simulink model "untitledlineal"  (R2014a)
settings: Solver=ode45  StartTime=0.0  StopTime=100  RelTol=1e-3
settings Model: Creator=Sec-E-B Ingenieria  LastModifiedBy=Sec-E-B Ingenieria

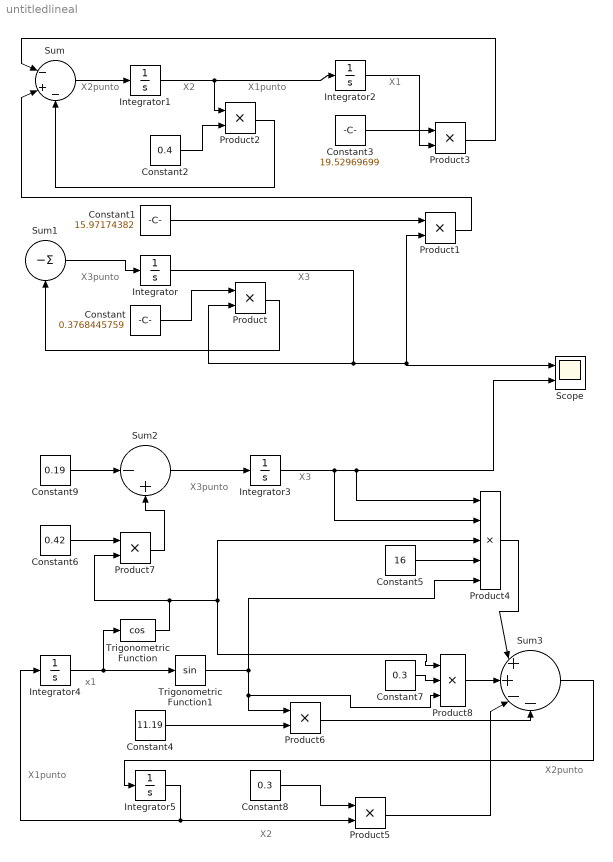
== system untitledlineal ==
  note: X3
  note: X3punto
  note: X1
  note: X1punto
  note: X2
  note: X2punto
  note: x1
  note: X1punto
  note: X2
  note: X2punto
  note: X3
  note: X3punto
  Constant : Constant  Value=0.3768445759
  Constant1 : Constant  Value=15.97174382
  Constant2 : Constant  Value=0.4
  Constant3 : Constant  Value=19.52969699
  Constant4 : Constant  Value=11.19
  Constant5 : Constant  Value=16
  Constant6 : Constant  Value=0.42
  Constant7 : Constant  Value=0.3
  Constant8 : Constant  Value=0.3
  Constant9 : Constant  Value=0.19
  Integrator : Integrator  InitialCondition=3
  Integrator1 : Integrator
  Integrator2 : Integrator
  Integrator3 : Integrator  InitialCondition=-1
  Integrator4 : Integrator  InitialCondition=1
  Integrator5 : Integrator
  Product{,1..3,5..7} (7 alike) : Product
  Product4 : Product  Inputs=5  InputSameDT=on
  Product8 : Product  Inputs=3
  Scope : Scope  NumInputPorts=2
      settings: YMin=-5~-5  YMax=5~5
  Sum : Sum  Inputs=|-+-
  Sum1 : Sum  Inputs=|-
  Sum2 : Sum  Inputs=|-+
  Sum3 : Sum  Inputs=|++--
  Trigonometric Function : Trigonometry  Operator=cos
  Trigonometric Function1 : Trigonometry
  wires:
  Sum1/1 -> Integrator/1
  Integrator/1 -> Product1/2, Scope/1, Product/2
  Product/1 -> Sum1/1
  Constant/1 -> Product/1
  Constant1/1 -> Product1/1
  Product1/1 -> Sum/2
  Sum/1 -> Integrator1/1
  Integrator1/1 -> Product2/1, Integrator2/1
  Constant2/1 -> Product2/2
  Product3/1 -> Sum/1
  Product2/1 -> Sum/3
  Sum2/1 -> Integrator3/1
  Integrator3/1 -> Product4/2, Scope/2, Product4/1
  Integrator4/1 -> Trigonometric Function1/1, Trigonometric Function/1
  Product4/1 -> Sum3/1
  Trigonometric Function1/1 -> Product4/5, Product6/1, Product8/3
  Constant4/1 -> Product6/2
  Trigonometric Function/1 -> Product8/1, Product4/3, Product7/2
  Product6/1 -> Sum3/4
  Sum3/1 -> Integrator5/1
  Integrator5/1 -> Product5/2, Integrator4/1
  Constant6/1 -> Product7/1
  Product7/1 -> Sum2/2
  Constant7/1 -> Product8/2
  Product8/1 -> Sum3/2
  Constant5/1 -> Product4/4
  Product5/1 -> Sum3/3
  Constant9/1 -> Sum2/1
  Constant8/1 -> Product5/1
  Integrator2/1 -> Product3/2
  Constant3/1 -> Product3/1
